simulink model "sdruFMMonoFPGAretarget"  (Simulink 8.1)
settings: Solver=FixedStepDiscrete  SolverMode=SingleTasking  StartTime=0.0  StopTime=inf  RelTol=1e-3
PreLoadFcn:
  | monoFM = getParamsSdruFMMonoDemo;
InitFcn:
  | monoFM = getParamsSdruFMMonoDemo;
undefined symbols (not defined in the file or in its folder): mfilt
libraries: simulink x1, dspmlti4 x1, dsparch4 x1, dspsnks4 x1, sdrublksprivate x1, commsdrhw_v2 x1
Description:
  | This model uses the Universal Software Radio Peripheral 2 (USRP2) device with Simulink(R) to perform FM mono demodulation.
CloseFcn:
  | clear monoFM
settings Model: Creator=The MathWorks Inc.  SimulationMode=rapid-accelerator
settings DataIOCC: SaveOutput=off  SignalLogging=off  DSMLogging=off  SaveTime=off
settings OptimizationCC: SimCompilerOptimization=On
settings DebuggingCC: InheritedTsInSrcMsg=none  MultiTaskCondExecSysMsg=none  ParameterPrecisionLossMsg=none
settings SFSimCC: SFSimEnableDebug=off  SFSimOverflowDetection=off  SimIntegrity=off
settings RTWCC: CustomSourceCode=|
  | #include<stdio.h>
  | #include<stdlib.h>

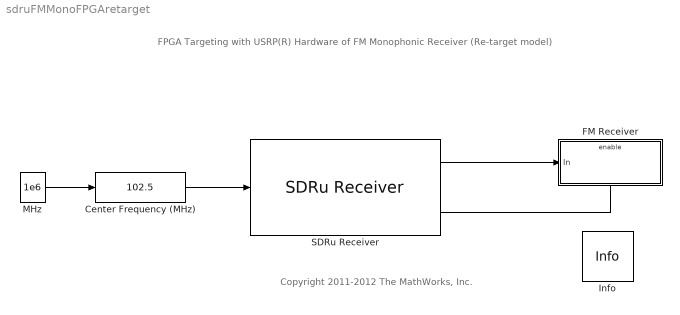
== system sdruFMMonoFPGAretarget ==
  note: Copyright 2011-2012 The MathWorks, Inc.
  note: FPGA Targeting with USRP(R) Hardware of FM Monophonic Receiver
      | (Re-target model)
  Center Frequency (MHz) : simulink/Math Operations/Slider Gain  low=87.5  gain=102.5  high=108
  FM Receiver : Subsystem  TreatAsAtomicUnit=on
  Info : sdrublksprivate/Info  SystemSampleTime=-1
  MHz : Constant  Value=1e6  VectorParams1D=off  SampleTime=-1  FramePeriod=-1
  SDRu Receiver : commsdrhw_v2/SDRu Receiver  rxtx=rx  USRP2_IP='192.168.10.2'  centerFrequency=2.45e9  centerFrequencySrc=Input port  loOffset=0  loOffsetSrc=Dialog  gain=monoFM.USRPGaindB  gainSrc=Dialog  decimInterp=monoFM.USRPDecimationFactor  decimInterpSrc=Dialog  USRP2_IP_NUM=[49 57 50 46 49 54 56 46 49 48 46 50]  frameLength=monoFM.FrameLength  outputDatatype=int16  overrunUnderrunPort=off  sampleTime=1/monoFM.Fs  HOST_DATA_PORT=30000  HOST_CONTROL_PORT=30002  USRP2_DATA_PORT=32769  USRP2_CONTROL_PORT=32768  bufferMode=Continuous streaming  EnableBurstMode=off  NumFramesInBurst=100
  wires:
  Center Frequency (MHz)/1 -> SDRu Receiver/1
  SDRu Receiver/2 -> FM Receiver/Enable
  MHz/1 -> Center Frequency (MHz)/1
  SDRu Receiver/1 -> FM Receiver/1(In)

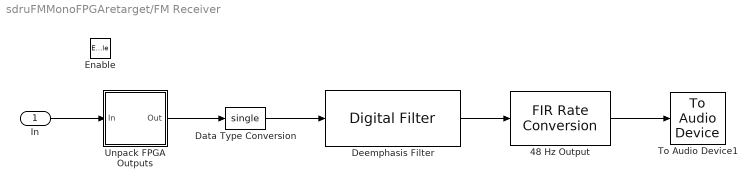
== system sdruFMMonoFPGAretarget/FM Receiver ==
  In : Inport
  Enable : EnablePort
  48 Hz Output : dspmlti4/FIR Rate Conversion  L=monoFM.InterpolationFactor  h=monoFM.Lowpass15k  M=monoFM.DecimationFactor  firstCoeffDataTypeStr=Inherit: Same word length as input  firstCoeffLastDataTypeStr=Inherit: Same word length as input  firstCoeffMin=[]  firstCoeffMax=[]  outputDataTypeStr=Inherit: Same as accumulator  outputLastDataTypeStr=Inherit: Same as accumulator  outputMin=[]  outputMax=[]  roundingMode=Floor  overflowMode=off  FilterSource=Specify via dialog  FilterObject=mfilt.firsrc(6,5)
  Data Type Conversion : DataTypeConversion  OutDataTypeStr=single
  Deemphasis Filter : dsparch4/Digital Filter  TypePopup=IIR (poles & zeros)  IIRFiltStruct=Direct form II transposed  AllPoleFiltStruct=Direct form  FIRFiltStruct=Direct form  CoeffSource=Specify via dialog  NumCoeffs=[1 2]  DenCoeffs=[1 0.1]  BiQuadCoeffs=[1 0.3 0.4 1 0.1 0.2]  LatticeCoeffs=[0.2 0.4]  denIgnore=on  FiltPerSampPopup=One filter per frame  IC=0  ICnum=0  ICden=0  roundingMode=Floor  overflowMode=off  ScaleValues=1  scaleValueFracLength=14  stageInFracLength=15  stageOutFracLength=15  FilterSource=dfilt object  dfiltObjectName=monoFM.DeemphasisFilter  InputProcessing=Columns as channels (frame based)
  To Audio Device1 : dspsnks4/To Audio Device  deviceName=Default  inheritSampleRate=on  sampleRate=48009  deviceDatatype=Determine from input data type  autoBufferSize=on  bufferSize=4096  queueDuration=1.0
  Unpack FPGA Outputs : Subsystem
  wires:
  Deemphasis Filter/1 -> 48 Hz Output/1
  48 Hz Output/1 -> To Audio Device1/1
  Unpack FPGA Outputs/1(Out) -> Data Type Conversion/1
  Data Type Conversion/1 -> Deemphasis Filter/1
  In/1 -> Unpack FPGA Outputs/1(In)

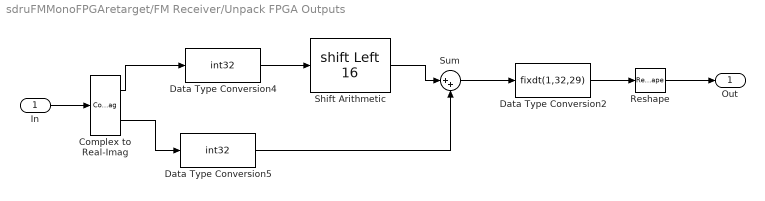
== system sdruFMMonoFPGAretarget/FM Receiver/Unpack FPGA Outputs ==
  In : Inport
  Complex to Real-Imag : ComplexToRealImag
  Data Type Conversion2 : DataTypeConversion  OutDataTypeStr=fixdt(1,32,29)  ConvertRealWorld=Stored Integer (SI)
  Data Type Conversion4 : DataTypeConversion  OutDataTypeStr=int32  ConvertRealWorld=Stored Integer (SI)
  Data Type Conversion5 : DataTypeConversion  OutDataTypeStr=int32  ConvertRealWorld=Stored Integer (SI)
  Reshape : Reshape  OutputDimensionality=Column vector (2-D)
  Shift Arithmetic : ArithShift  BitShiftNumber=16  BitShiftDirection=Left
  Sum : Sum  Inputs=|++  OutDataTypeStr=int32
  Out : Outport
  wires:
  Shift Arithmetic/1 -> Sum/1
  Sum/1 -> Data Type Conversion2/1
  Data Type Conversion4/1 -> Shift Arithmetic/1
  Data Type Conversion5/1 -> Sum/2
  Data Type Conversion2/1 -> Reshape/1
  Complex to Real-Imag/2 -> Data Type Conversion5/1
  Reshape/1 -> Out/1
  Complex to Real-Imag/1 -> Data Type Conversion4/1
  In/1 -> Complex to Real-Imag/1
